simulink model "MdEnAndBsySelc"  (R2018b)
settings: Solver=FixedStepDiscrete  StartTime=0.0  StopTime=10.0  FixedStep=0.01  RelTol=1e-3
settings Model: Creator=sn2xws  LastModifiedBy=sn2xws
settings DataIOCC: SaveFormat=StructureWithTime
settings OptimizationCC: DefaultParameterBehavior=Inlined  EnhancedBackFolding=on  PassReuseOutputArgsAs=Individual arguments  ZeroExternalMemoryAtStartup=off  ZeroInternalMemoryAtStartup=off  OptimizeBlockOrder=speed  DifferentSizesBufferReuse=on  OptimizationCustomize=off
settings DebuggingCC: ParameterTunabilityLossMsg=error
settings ModelReferenceCC: ModelReferenceNumInstancesAllowed=Single
settings SFSimCC: MATLABDynamicMemAlloc=off
settings RTWCC: SystemTargetFile=autosar.tlc  GenCodeOnly=on  TemplateMakefile=ert_default_tmf  Description=AUTOSAR  GenerateReport=on  IncludeHyperlinkInReport=on  LaunchReport=on  GenerateTraceInfo=on  GenerateTraceReport=on  GenerateTraceReportSl=on  GenerateTraceReportSf=on  GenerateTraceReportEml=on  GenerateCodeMetricsReport=on
settings CodeAppCC: ForceParamTrailComments=on  IgnoreCustomStorageClasses=off  OperatorAnnotations=on  SimulinkDataObjDesc=on  SFDataObjDesc=on  InsertBlockDesc=on
settings STFCustomTargetCC: TargetLangStandard=C99 (ISO)  MultiwordLength=256  ParMdlRefBuildCompliant=on  CompOptLevelCompliant=on  IncludeMdlTerminateFcn=off  CombineOutputUpdateFcns=on  SuppressErrorStatus=on  ERTCustomFileBanners=on  SupportNonFinite=off  SupportComplex=off  SupportContinuousTime=off  SupportNonInlinedSFcns=off  RemoveResetFunc=on  MATLABClassNameForMDSCustomization=Simulink.SoftwareTarget.ERTCustomization  AutosarCompliant=on  UseToolchainInfoCompliant=on  LookupTableObjectStructAxisOrder=2,1,3,4,...  LUTObjectStructOrderEvenSpacing=Size,Table,Breakpoints  SystemTargetFile=autosar.tlc
settings ERTTargetCC: TargetLangStandard=C99 (ISO)  ConcurrentExecutionCompliant=off  IncludeMdlTerminateFcn=off  SuppressErrorStatus=on  SupportNonFinite=off  SupportComplex=off  ModelStepFunctionPrototypeControlCompliant=off  CPPClassGenCompliant=off  AutosarCompliant=on  LookupTableObjectStructAxisOrder=2,1,3,4,...  LUTObjectStructOrderEvenSpacing=Size,Table,Breakpoints  InlinedParameterPlacement=NonHierarchical  ERTCustomFileTemplate=example_file_process.tlc

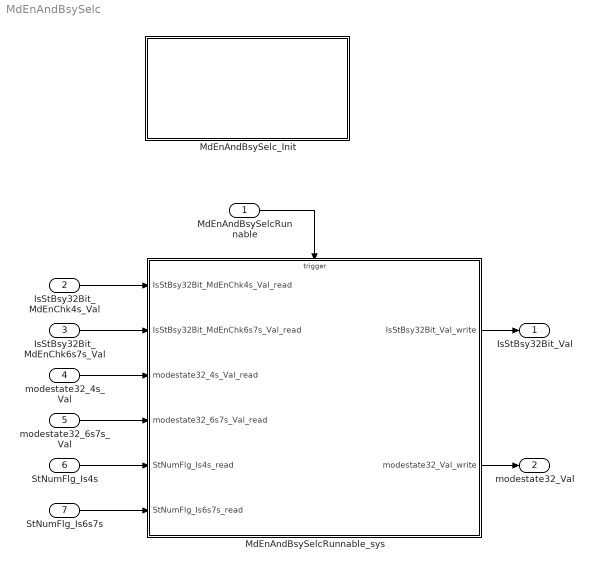
== system MdEnAndBsySelc ==
  MdEnAndBsySelcRunnable : Inport  SampleTime=0.01  OutputFunctionCall=on
  IsStBsy32Bit_MdEnChk4s_Val : Inport  Port=2  OutDataTypeStr=uint32  PortDimensions=1
  IsStBsy32Bit_MdEnChk6s7s_Val : Inport  Port=3  OutDataTypeStr=uint32  PortDimensions=1
  modestate32_4s_Val : Inport  Port=4  OutDataTypeStr=uint32  PortDimensions=1
  modestate32_6s7s_Val : Inport  Port=5  OutDataTypeStr=uint32  PortDimensions=1
  StNumFlg_Is4s : Inport  Port=6  OutDataTypeStr=boolean  PortDimensions=1
  StNumFlg_Is6s7s : Inport  Port=7  OutDataTypeStr=boolean  PortDimensions=1
  MdEnAndBsySelcRunnable_sys : Subsystem
  MdEnAndBsySelc_Init : Subsystem
  IsStBsy32Bit_Val : Outport  OutDataTypeStr=uint32  PortDimensions=1
  modestate32_Val : Outport  Port=2  OutDataTypeStr=uint32  PortDimensions=1
  wires:
  IsStBsy32Bit_MdEnChk4s_Val/1 -> MdEnAndBsySelcRunnable_sys/1(IsStBsy32Bit_MdEnChk4s_Val_read)
  IsStBsy32Bit_MdEnChk6s7s_Val/1 -> MdEnAndBsySelcRunnable_sys/2(IsStBsy32Bit_MdEnChk6s7s_Val_read)
  modestate32_4s_Val/1 -> MdEnAndBsySelcRunnable_sys/3(modestate32_4s_Val_read)
  modestate32_6s7s_Val/1 -> MdEnAndBsySelcRunnable_sys/4(modestate32_6s7s_Val_read)
  StNumFlg_Is4s/1 -> MdEnAndBsySelcRunnable_sys/5(StNumFlg_Is4s_read)
  StNumFlg_Is6s7s/1 -> MdEnAndBsySelcRunnable_sys/6(StNumFlg_Is6s7s_read)
  MdEnAndBsySelcRunnable_sys/1(IsStBsy32Bit_Val_write) -> IsStBsy32Bit_Val/1
  MdEnAndBsySelcRunnable_sys/2(modestate32_Val_write) -> modestate32_Val/1
  MdEnAndBsySelcRunnable/1 -> MdEnAndBsySelcRunnable_sys/Trigger

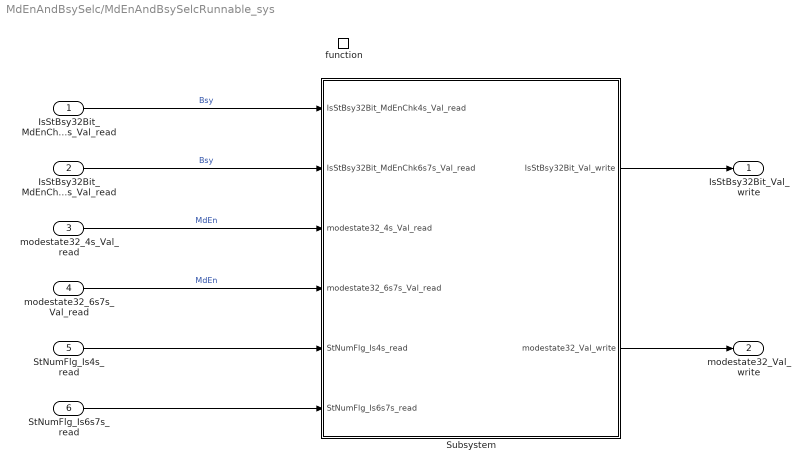
== system MdEnAndBsySelc/MdEnAndBsySelcRunnable_sys ==
  IsStBsy32Bit_MdEnChk4s_Val_read : Inport
  IsStBsy32Bit_MdEnChk6s7s_Val_read : Inport  Port=2
  modestate32_4s_Val_read : Inport  Port=3
  modestate32_6s7s_Val_read : Inport  Port=4
  StNumFlg_Is4s_read : Inport  Port=5
  StNumFlg_Is6s7s_read : Inport  Port=6
  function : TriggerPort  TriggerType=function-call  VariantControl=(inherit)  SampleTimeType=periodic  SampleTime=-1
  Subsystem : Subsystem
  IsStBsy32Bit_Val_write : Outport
      settings: EnsureOutportIsVirtual=on
  modestate32_Val_write : Outport  Port=2
      settings: EnsureOutportIsVirtual=on
  wires:
  IsStBsy32Bit_MdEnChk4s_Val_read/1 -> Subsystem/1(IsStBsy32Bit_MdEnChk4s_Val_read)  "Bsy"
  IsStBsy32Bit_MdEnChk6s7s_Val_read/1 -> Subsystem/2(IsStBsy32Bit_MdEnChk6s7s_Val_read)  "Bsy"
  modestate32_4s_Val_read/1 -> Subsystem/3(modestate32_4s_Val_read)  "MdEn"
  modestate32_6s7s_Val_read/1 -> Subsystem/4(modestate32_6s7s_Val_read)  "MdEn"
  StNumFlg_Is4s_read/1 -> Subsystem/5(StNumFlg_Is4s_read)
  StNumFlg_Is6s7s_read/1 -> Subsystem/6(StNumFlg_Is6s7s_read)
  Subsystem/1(IsStBsy32Bit_Val_write) -> IsStBsy32Bit_Val_write/1
  Subsystem/2(modestate32_Val_write) -> modestate32_Val_write/1

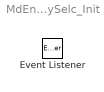
== system MdEnAndBsySelc/MdEnAndBsySelc_Init ==
  Event Listener : EventListener  EventName=reset

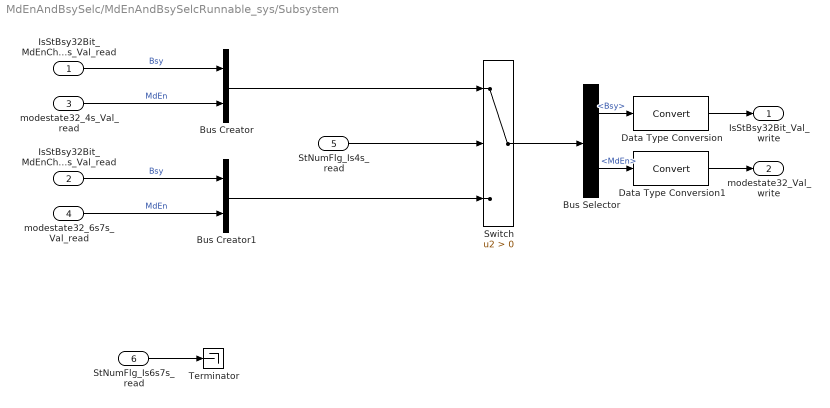
== system MdEnAndBsySelc/MdEnAndBsySelcRunnable_sys/Subsystem ==
  IsStBsy32Bit_MdEnChk4s_Val_read : Inport
  IsStBsy32Bit_MdEnChk6s7s_Val_read : Inport  Port=2
  modestate32_4s_Val_read : Inport  Port=3
  modestate32_6s7s_Val_read : Inport  Port=4
  StNumFlg_Is4s_read : Inport  Port=5
  StNumFlg_Is6s7s_read : Inport  Port=6
  Bus Creator : BusCreator  Inputs=2
  Bus Creator1 : BusCreator  Inputs=2
  Bus Selector : BusSelector  OutputSignals=Bsy,MdEn
  Data Type Conversion : DataTypeConversion
  Data Type Conversion1 : DataTypeConversion
  Switch : Switch  Criteria=u2 > Threshold
  Terminator : Terminator
  IsStBsy32Bit_Val_write : Outport
      settings: EnsureOutportIsVirtual=on
  modestate32_Val_write : Outport  Port=2
      settings: EnsureOutportIsVirtual=on
  wires:
  Bus Creator/1 -> Switch/1
  modestate32_4s_Val_read/1 -> Bus Creator/2  "MdEn"
  IsStBsy32Bit_MdEnChk4s_Val_read/1 -> Bus Creator/1  "Bsy"
  Bus Creator1/1 -> Switch/3
  Bus Selector/1 -> Data Type Conversion/1  "<Bsy>"
  Bus Selector/2 -> Data Type Conversion1/1  "<MdEn>"
  Switch/1 -> Bus Selector/1
  StNumFlg_Is4s_read/1 -> Switch/2
  StNumFlg_Is6s7s_read/1 -> Terminator/1
  Data Type Conversion/1 -> IsStBsy32Bit_Val_write/1
  Data Type Conversion1/1 -> modestate32_Val_write/1
  modestate32_6s7s_Val_read/1 -> Bus Creator1/2  "MdEn"
  IsStBsy32Bit_MdEnChk6s7s_Val_read/1 -> Bus Creator1/1  "Bsy"
